simulink model "Localization_Model"  (R2015a)
settings: Solver=ode45  StartTime=0.0  StopTime=10.0  RelTol=1e-3
settings Model: Creator=Bruno  LastModifiedBy=David

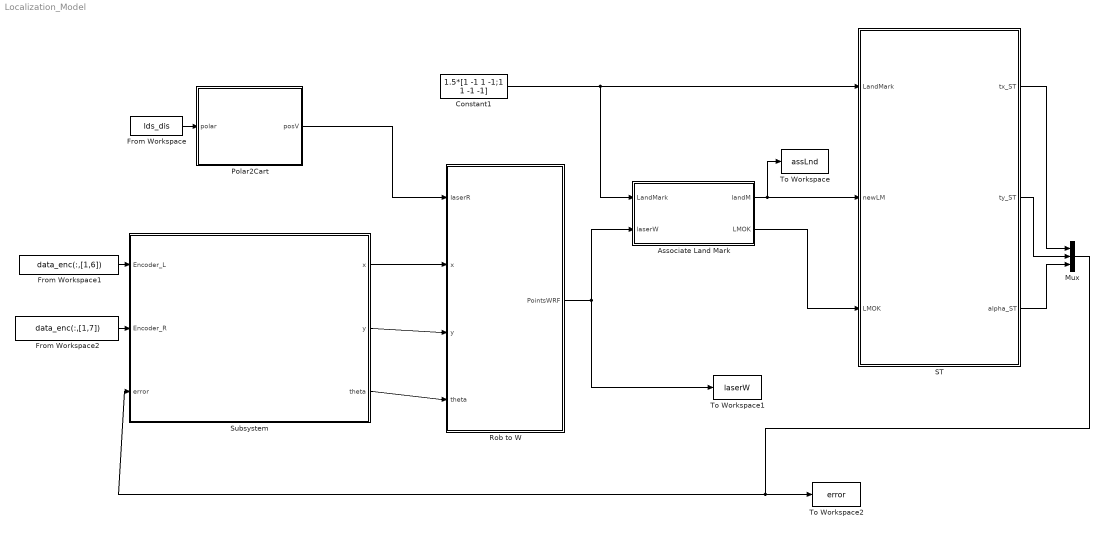
== system Localization_Model ==
  Associate Land Mark : MATLAB Function  TreatAsAtomicUnit=on
  Constant1 : Constant  Value=1.5*[1 -1 1 -1;1 1 -1 -1]
  From Workspace : FromWorkspace  VariableName=lds_dis  SampleTime=0
  From Workspace1 : FromWorkspace  VariableName=data_enc(:,[1,6])  SampleTime=0
  From Workspace2 : FromWorkspace  VariableName=data_enc(:,[1,7])  SampleTime=0
  Mux : Mux  Inputs=3
  Polar2Cart : MATLAB Function  TreatAsAtomicUnit=on
  Rob to W : MATLAB Function  TreatAsAtomicUnit=on
  ST : MATLAB Function  TreatAsAtomicUnit=on
  Subsystem : Subsystem
  To Workspace : ToWorkspace  VariableName=assLnd  SaveFormat=Timeseries  SampleTime=-1
  To Workspace1 : ToWorkspace  VariableName=laserW  SaveFormat=Timeseries  SampleTime=-1
  To Workspace2 : ToWorkspace  VariableName=error  SaveFormat=Timeseries  SampleTime=-1
  wires:
  Polar2Cart/1(posV) -> Rob to W/1(laserR)
  Constant1/1 -> Associate Land Mark/1(LandMark), ST/1(LandMark)
  Associate Land Mark/1(landM) -> To Workspace/1, ST/2(newLM)
  Rob to W/1(PointsWRF) -> To Workspace1/1, Associate Land Mark/2(laserW)
  ST/1(tx_ST) -> Mux/1
  Subsystem/1(x) -> Rob to W/2(x)
  Subsystem/2(y) -> Rob to W/3(y)
  Subsystem/3(theta) -> Rob to W/4(theta)
  From Workspace/1 -> Polar2Cart/1(polar)
  From Workspace2/1 -> Subsystem/2(Encoder_R)
  From Workspace1/1 -> Subsystem/1(Encoder_L)
  Associate Land Mark/2(LMOK) -> ST/3(LMOK)
  ST/2(ty_ST) -> Mux/2
  ST/3(alpha_ST) -> Mux/3
  Mux/1 -> To Workspace2/1, Subsystem/3(error)

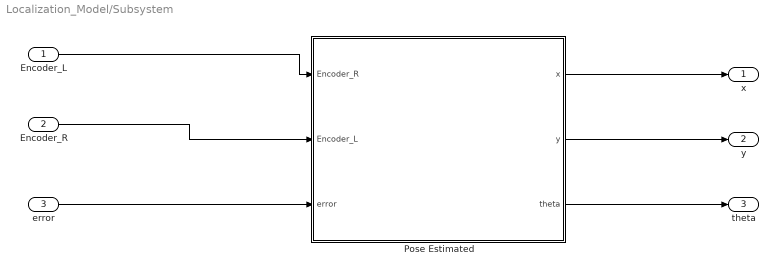
== system Localization_Model/Subsystem ==
  Encoder_L : Inport
  Encoder_R : Inport  Port=2
  error : Inport  Port=3
  Pose Estimated : MATLAB Function  TreatAsAtomicUnit=on
  x : Outport
  y : Outport  Port=2
  theta : Outport  Port=3
  wires:
  Encoder_L/1 -> Pose Estimated/1(Encoder_R)
  Encoder_R/1 -> Pose Estimated/2(Encoder_L)
  error/1 -> Pose Estimated/3(error)
  Pose Estimated/3(theta) -> theta/1
  Pose Estimated/2(y) -> y/1
  Pose Estimated/1(x) -> x/1

== matlab function Localization_Model/Rob to W ==
  data: laserR input; PointsWRF output; x input; y input; theta input
function PointsWRF = rob2W(laserR,x,y,theta)
    
    laserR = [laserR;zeros(1,360);ones(1,360)];
    PointsWRF = transl(x,y,0)*trotz(theta)*laserR;
    PointsWRF = PointsWRF(1:2,:);

end

== matlab function Localization_Model/Polar2Cart ==
  data: polar input; posV output
function posV = polar2Cart(polar)

    angle = 1:360;
    angle = angle*2*pi/360;
    lx = polar'.*cos(angle)/1000;
    ly = polar'.*sin(angle)/1000;
    
    posV = [lx;ly];
end

== matlab function Localization_Model/Associate Land Mark ==
  data: LandMark input; landM output; laserW input; LMOK output
function [landM,LMOK] = assoLndMrk(LandMark,laserW)

    lx=laserW(1,:);
    ly=laserW(2,:);
    landM=[];
    LMOK=ones(1,4);
    for i=1:4 %Group the laser if they are near or far from the LM
       distLM=sqrt((lx-LandMark(1,i)).^2+(ly-LandMark(2,i)).^2);
       goodL=[lx(distLM<distTH);ly(distLM<distTH)];
       if length(goodL)>2
           landM=[landM mean(goodL')'];
       else
           LMOK(i)=0;
       end
    end

== matlab function Localization_Model/ST ==
  data: LandMark input; newLM input; tx_ST output; LMOK input; ty_ST output; alpha_ST output
function [tx_ST,ty_ST,alpha_ST] = ST(LandMark,newLM,LMOK)
    if length(newLM)>1
        LandMark=LandMark(:,LMOK==1);
        A =zeros(2*sum(LMOK),4);
        for i=1:sum(LMOK)
            A(2*i-1,:) = [LandMark(1,i),LandMark(2,i),1,0];
            A(2*i-1,:) = [LandMark(2,i),-LandMark(1,i),0,1];
        end
        B = zeros(2*sum(LMOK),1);%Build Matrix B
        for i=1:sum(LMOK)
            B(2*i-1:2*i) = [newLM(1,i); newLM(2,i)];
        end
        %Compute tx ty i tita
        X = inv((A'*A))*A'*B;
        tx_ST = X(3);
        ty_ST = X(4);
        alpha_ST = atan2(X(2),X(1));
    else
        tx_ST=0;
        ty_ST=0;
        alpha_ST=0;
    end
end

== matlab function Localization_Model/Subsystem/Pose Estimated ==
  data: Encoder_R input; x output; Encoder_L input; error input; y output; theta output
function [x,y,theta] = Pose_Est(Encoder_R,Encoder_L,error)
    
    %  internal variable to be mantain its values
    persistent x_w y_w suma_theta
    %  variable initialization
    if isempty (x_w)
        x_w=0;
    end
    if isempty (y_w)
        y_w=0;
    end
    if isempty (suma_theta)
        suma_theta=0;
    end
    %  compute the odometry    %
    delta_th=(Encoder_R-Encoder_L)/0.243;
    delta_d=(Encoder_L+Encoder_R)/2;
    %  integration of the robot pose %
    x_w=x_w + delta_d*cos(suma_theta)-error(1);
    y_w=y_w + delta_d*sin(suma_theta)-error(2);
    suma_theta=mod(suma_theta+delta_th-error(3),2*pi);
    %  output variable %
    x=x_w;
    y=y_w;
    theta=suma_theta;
  
end
